simulink model "tanksim"  (R2024a)
settings: Solver=VariableStepAuto  StartTime=0.0  StopTime=T  RelTol=1e-3
values from neighbouring files (symbols this model uses):
  A = 1    [init.m]
  h_0 = 0    [init.m]
  h_r = 0.5    [init.m]
  k = 1    [init.m]
  K_p = 100    [init.m]
  rho = 1000    [init.m]
settings Model: Creator=Lars André  LastModifiedBy=Lars André

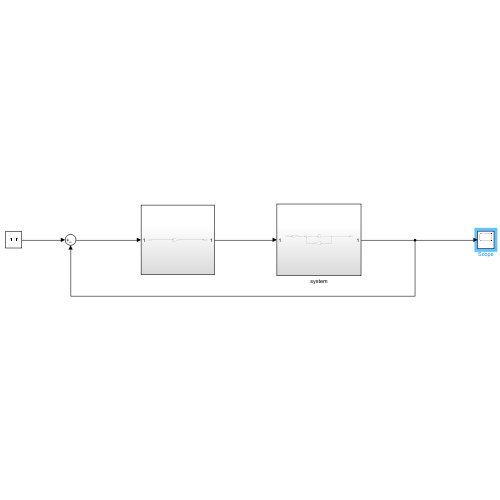
[thumbnail: Simulink's stored preview of the top-level diagram]
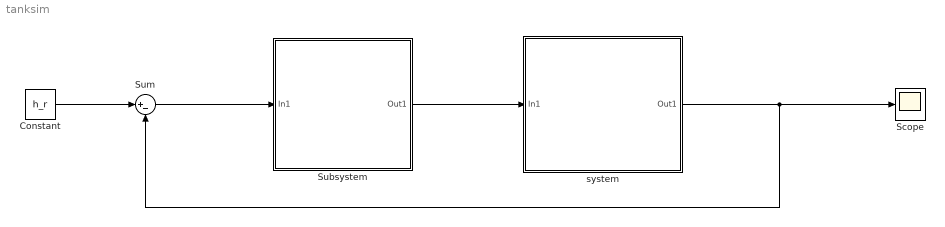
== system tanksim ==
  Constant : Constant  Value=h_r
  Scope : Scope
  Subsystem : Subsystem
  Sum : Sum  Inputs=|+-
  system : Subsystem
  wires:
  system/1(Out1) -> Sum/2, Scope/1
  Subsystem/1(Out1) -> system/1(In1)
  Sum/1 -> Subsystem/1(In1)
  Constant/1 -> Sum/1

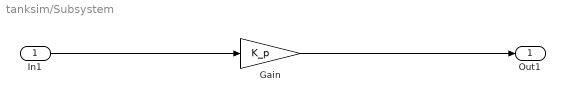
== system tanksim/Subsystem ==
  In1 : Inport
  Gain : Gain  Gain=K_p
  Out1 : Outport
  wires:
  Gain/1 -> Out1/1
  In1/1 -> Gain/1

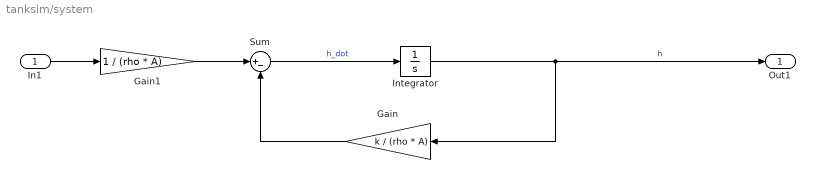
== system tanksim/system ==
  In1 : Inport
  Gain : Gain  Gain=k / (rho * A)
  Gain1 : Gain  Gain=1 / (rho * A)
  Integrator : Integrator  InitialCondition=h_0
  Sum : Sum  Inputs=|+-
  Out1 : Outport
  wires:
  Gain/1 -> Sum/2
  Sum/1 -> Integrator/1  "h_dot"
  Integrator/1 -> Out1/1, Gain/1  "h"
  In1/1 -> Gain1/1
  Gain1/1 -> Sum/1
